simulink subsystem "s1EM"  (R2024b)
settings: Solver=VariableStepAuto  StartTime=0.0  StopTime=10.0  RelTol=1e-3
undefined symbols (not defined in the file): PlntEMCp, PlntEMMass
libraries: autolibutils x1, autolibsharedcommon x1
settings Model: ModifiedByFormat=The MathWorks, Inc.  Creator=The MathWorks, Inc.  LastModifiedBy=The MathWorks, Inc.
settings RTWCC: GPUComputeCapability=3.5

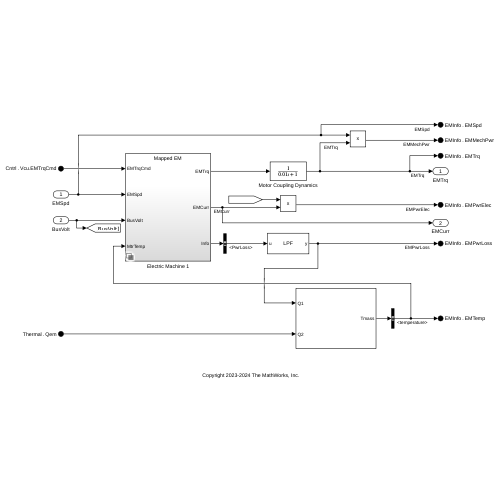
[thumbnail: Simulink's stored preview of the top-level diagram]
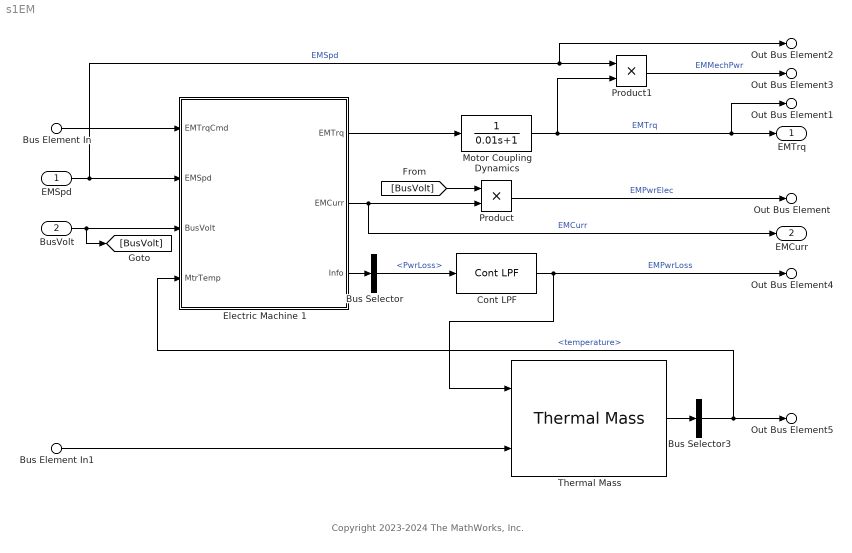
== system s1EM ==
  note: Copyright 2023-2024 The MathWorks, Inc.
  EMSpd : Inport
  BusVolt : Inport  Port=2
  Bus Element In : Inport  Port=3  PortName=Cntrl  Element=Vcu.EMTrqCmd
  Bus Element In1 : Inport  Port=4  PortName=Thermal  Element=Qem
  Bus Selector : BusSelector  OutputSignals=PwrLoss
  Bus Selector3 : BusSelector  OutputSignals=temperature
  Cont LPF : autolibutils/Cont LPF  wc=1  AbsoluteTolerance=auto  aMode=6
  Electric Machine 1 : Subsystem  Variant=on  VariantControlMode=label  LabelModeActiveChoice=Mapped EM
  Motor Coupling Dynamics : TransferFcn  Denominator=[0.01 1]
  Product : Product
  Product1 : Product
  Thermal Mass : autolibsharedcommon/Thermal Mass  MassOrVol=Mass  Mass=PlntEMMass  Volume=10  Rho=997  HeatCp=PlntEMCp*ones(1,2)  HeatBrkPts=PlntBattCpBpt  Tinit=EnvAirTemp  Tenv=EnvAirTemp  ConvHTC=1  EnvArea=0.1
  EMTrq : Outport
  EMCurr : Outport  Port=2
  Out Bus Element : Outport  Port=3  PortName=EMInfo  Element=EMPwrElec
  Out Bus Element1 : Outport  Port=3  PortName=EMInfo  Element=EMTrq
  Out Bus Element2 : Outport  Port=3  PortName=EMInfo  Element=EMSpd
  Out Bus Element3 : Outport  Port=3  PortName=EMInfo  Element=EMMechPwr
  Out Bus Element4 : Outport  Port=3  PortName=EMInfo  Element=EMPwrLoss
  Out Bus Element5 : Outport  Port=3  PortName=EMInfo  Element=EMTemp
  wires:
  Bus Element In/1 -> Electric Machine 1/1(EMTrqCmd)
  BusVolt/1 -> [BusVolt], Electric Machine 1/3(BusVolt)
  Product/1 -> Out Bus Element/1  "EMPwrElec"
  Electric Machine 1/2(EMCurr) -> EMCurr/1, Product/2  "EMCurr"
  Electric Machine 1/1(EMTrq) -> Motor Coupling Dynamics/1
  [BusVolt] -> Product/1
  Electric Machine 1/3(Info) -> Bus Selector/1
  Bus Element In1/1 -> Thermal Mass/2
  Cont LPF/1 -> Out Bus Element4/1, Thermal Mass/1  "EMPwrLoss"
  Bus Selector/1 -> Cont LPF/1  "<PwrLoss>"
  Thermal Mass/1 -> Bus Selector3/1
  Bus Selector3/1 -> Electric Machine 1/4(MtrTemp), Out Bus Element5/1  "<temperature>"
  Product1/1 -> Out Bus Element3/1  "EMMechPwr"
  Motor Coupling Dynamics/1 -> Product1/2, Out Bus Element1/1, EMTrq/1  "EMTrq"
  EMSpd/1 -> Out Bus Element2/1, Product1/1, Electric Machine 1/2(EMSpd)  "EMSpd"

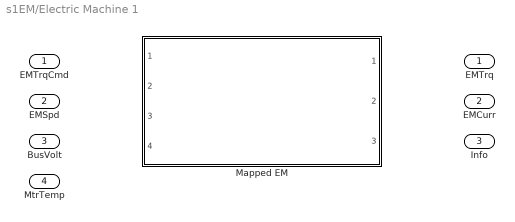
== system s1EM/Electric Machine 1 ==
  EMTrqCmd : Inport
  EMSpd : Inport  Port=2
  BusVolt : Inport  Port=3
  MtrTemp : Inport  Port=4
  Mapped EM : Subsystem  VariantControl=Mapped EM  ReferencedSubsystem=ElectricMachine1
  EMTrq : Outport  VectorParamsAs1DForOutWhenUnconnected=off
  EMCurr : Outport  Port=2  VectorParamsAs1DForOutWhenUnconnected=off
  Info : Outport  Port=3
